simulink model "F_to_tau"  (R2018a)
settings: Solver=VariableStepAuto  StartTime=0.0  StopTime=10.0  RelTol=1e-3
settings Model: Creator=MJ  LastModifiedBy=MJ

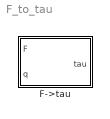
== system F_to_tau ==
  F->tau : MATLAB Function  TreatAsAtomicUnit=on

== matlab function F_to_tau/F->tau ==
  data: F input; tau output; q input
function tau = fcn(F,q)

q1 = q(1);
q2 = q(2);

J = reshape([ -(16695324718374375*cos(q1) - 2251799813685248*2^(1/2)*sin(q1))/(450359962737049600*((sin(q1)/10 - 3339064943674875/9007199254740992)^2 + (cos(q1)/10 - 2^(1/2)/20)^2)^(1/2)),                                                                                                                                                                             0]
[                                                                                                                                                                             0, -(16695324718374375*cos(q2) - 2251799813685248*2^(1/2)*sin(q2))/(450359962737049600*((sin(q2)/10 - 3339064943674875/9007199254740992)^2 + (cos(q2)/10 - 2^(1/2)/20)^2)^(1/2))],[2,2]);

tau = -J'*F;
